simulink model "Gardner"  (R2019b)
settings: Solver=VariableStepAuto  StartTime=0.0  StopTime=5e-3  RelTol=1e-3
values from neighbouring files (symbols this model uses):
  b = double(b)    [loopFil.m]
  filter = rcosdesign(alpha,symNum,sym,'sqrt')    [loopFil.m]
  G = 64    [loopFil.m]
libraries: dspsigops x5, dspsrcs4 x1
settings Model: Creator=Administrator  LastModifiedBy=Administrator

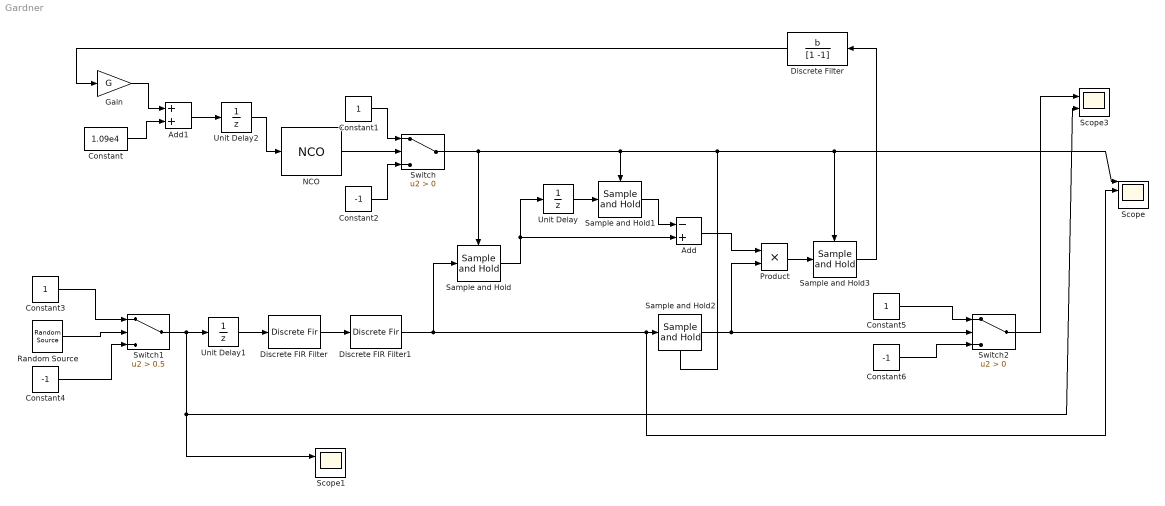
== system Gardner ==
  Add : Sum  Inputs=-+
  Add1 : Sum  OutDataTypeStr=int16
  Constant : Constant  Value=1.09e4  OutDataTypeStr=int32  SampleTime=1/(6*19.2e3)
  Constant1 : Constant  SampleTime=1/(6*19.2e3)
  Constant2 : Constant  Value=-1  SampleTime=1/(6*19.2e3)
  Constant3 : Constant  SampleTime=1/(6*19.2e3)
  Constant4 : Constant  Value=-1  SampleTime=1/(6*19.2e3)
  Constant5 : Constant  SampleTime=1/(6*19.2e3)
  Constant6 : Constant  Value=-1  SampleTime=1/(6*19.2e3)
  Discrete FIR Filter : DiscreteFir  Coefficients=filter
  Discrete FIR Filter1 : DiscreteFir  Coefficients=filter
  Discrete Filter : DiscreteFilter  Numerator=b  Denominator=[1 -1]  a0EqualsOne=on
  Gain : Gain  Gain=G
  NCO : dspsigops/NCO  AccIncSrc=Input port  AccInc=100  PhaseOffsetSrc=Specify via dialog  PhaseOffset=0  AccumWL=16  HasDither=on  DitherWL=4  PNgeneratorLength=19  HasPhaseQuantizer=on  TableDepth=12  HasOutputPhaseError=off  Formula=Sine  DataType=single  OutputWL=16  OutputFL=14  CompMethod=Table lookup (no interpolation)  SampleTime=1  SamplesPerFrame=1  OutputFrames=off
      settings: SourceProductName=DSP System Toolbox  SourceProductBaseCode=DS
  Product : Product
  Random Source : dspsrcs4/Random Source  SrcType=Uniform  NormMethod=Ziggurat  CltLength=12  MinVal=0  MaxVal=1  MeanVal=0  VarVal=1  RepMode=Not repeatable  rawSeed=1  IsInherit=off  SampMode=Discrete  SampTime=1/(19.2e3)  SampFrame=1  DataType=Double  OutComplex=Real  OutputFrames=off
  Sample and Hold : dspsigops/Sample and Hold  trig=Rising edge  initCond=0  latchinput=off
  Sample and Hold1 : dspsigops/Sample and Hold  trig=Rising edge  initCond=0  latchinput=off
  Sample and Hold2 : dspsigops/Sample and Hold  trig=Falling edge  initCond=0  latchinput=off
  Sample and Hold3 : dspsigops/Sample and Hold  Tag=error  trig=Rising edge  initCond=0  latchinput=off
  Scope : Scope  NumInputPorts=4
  Scope1 : Scope  NumInputPorts=2
  Scope3 : Scope  NumInputPorts=2
  Switch : Switch  Criteria=u2 > Threshold
  Switch1 : Switch  Criteria=u2 > Threshold  Threshold=0.5
  Switch2 : Switch  Criteria=u2 > Threshold
  Unit Delay : UnitDelay  SampleTime=-1  HasFrameUpgradeWarning=on
  Unit Delay1 : UnitDelay  SampleTime=-1  HasFrameUpgradeWarning=on
  Unit Delay2 : UnitDelay  SampleTime=-1  HasFrameUpgradeWarning=on
  wires:
  NCO/1 -> Switch/2
  Constant1/1 -> Switch/1
  Constant2/1 -> Switch/3
  Switch/1 -> Scope/1, Sample and Hold3/Trigger, Sample and Hold2/Trigger, Sample and Hold1/Trigger, Sample and Hold/Trigger
  Sample and Hold/1 -> Unit Delay/1, Add/2
  Unit Delay/1 -> Sample and Hold1/1
  Sample and Hold1/1 -> Add/1
  Add/1 -> Product/1
  Sample and Hold2/1 -> Switch2/2, Product/2
  Switch1/1 -> Scope1/1, Scope3/2, Unit Delay1/1
  Constant3/1 -> Switch1/1
  Unit Delay1/1 -> Discrete FIR Filter/1
  Random Source/1 -> Switch1/2
  Constant4/1 -> Switch1/3
  Product/1 -> Sample and Hold3/1
  Add1/1 -> Unit Delay2/1
  Gain/1 -> Add1/1
  Constant/1 -> Add1/2
  Unit Delay2/1 -> NCO/1
  Sample and Hold3/1 -> Discrete Filter/1
  Discrete Filter/1 -> Gain/1
  Constant5/1 -> Switch2/1
  Constant6/1 -> Switch2/3
  Switch2/1 -> Scope3/1
  Discrete FIR Filter/1 -> Discrete FIR Filter1/1
  Discrete FIR Filter1/1 -> Scope/2, Sample and Hold2/1, Sample and Hold/1
